simulink model "MODEL_joy"  (R2021a)
settings: Solver=VariableStepAuto  StartTime=0.0  StopTime=inf  RelTol=1e-3
undefined symbols (not defined in the file or in its folder): aircraft, Earth, FandM, MAV, plotprob, u_trim, WGS84
libraries: aerolibfltsims x2, aerolibanimutils x1, aerolibtransform2 x1
settings Model: Creator=DELL  LastModifiedBy=DELL

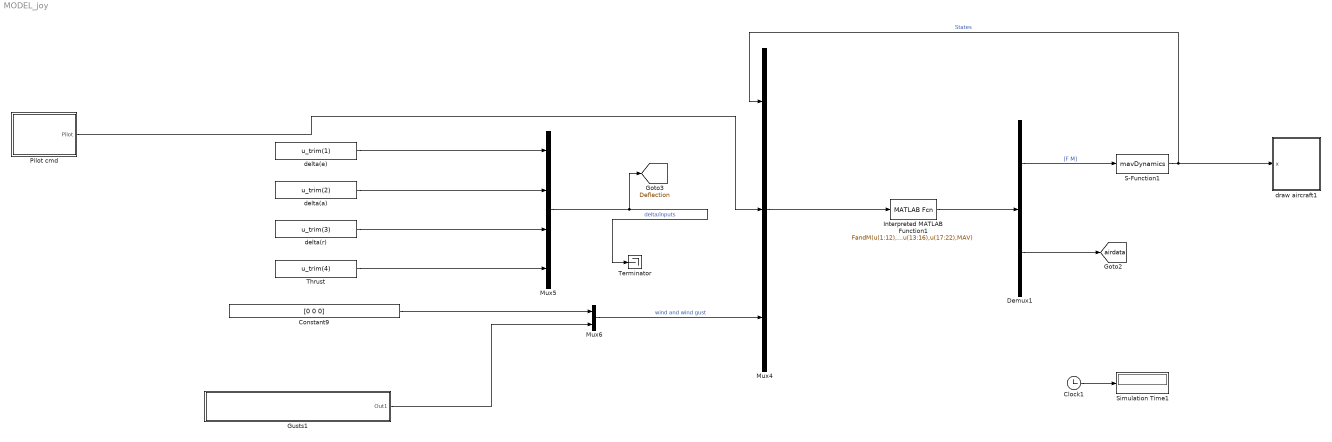
== system MODEL_joy ==
  Clock1 : Clock
  Constant9 : Constant  Value=[0 0 0]
  Demux1 : Demux  Outputs=[6;6]
  Gusts1 : Subsystem
  Interpreted MATLAB Function1 : MATLABFcn  MATLABFcn=FandM(u(1:12),u(13:16),u(17:22),MAV)  OutputDimensions=12
  Mux4 : Mux  Inputs=3
  Mux5 : Mux
  Mux6 : Mux  Inputs=2
  Pilot cmd : Subsystem
  S-Function1 : S-Function  FunctionName=mavDynamics  Parameters=MAV  SFunctionDeploymentMode=off  EnableBusSupport=off
  Simulation Time1 : Display
  Terminator : Terminator
  Thrust : Constant  Value=u_trim(4)
  delta(a) : Constant  Value=u_trim(2)
  delta(e) : Constant  Value=u_trim(1)
  delta(r) : Constant  Value=u_trim(3)
  draw aircraft1 : Subsystem
  tag scope: Deflection=global, airdata=global
  wires:
  Mux6/1 -> Mux4/3  "wind and wind gust"
  Demux1/2 -> [airdata]
  Constant9/1 -> Mux6/1
  Mux5/1 -> Terminator/1, [Deflection]  "delta/inputs"
  Clock1/1 -> Simulation Time1/1
  Mux4/1 -> Interpreted MATLAB Function1/1
  Interpreted MATLAB Function1/1 -> Demux1/1
  S-Function1/1 -> draw aircraft1/1(x), Mux4/1  "States"
  Gusts1/1(Out1) -> Mux6/2
  Demux1/1 -> S-Function1/1  "[F M]"
  delta(e)/1 -> Mux5/1
  delta(a)/1 -> Mux5/2
  delta(r)/1 -> Mux5/3
  Thrust/1 -> Mux5/4
  Pilot cmd/1(Pilot) -> Mux4/2

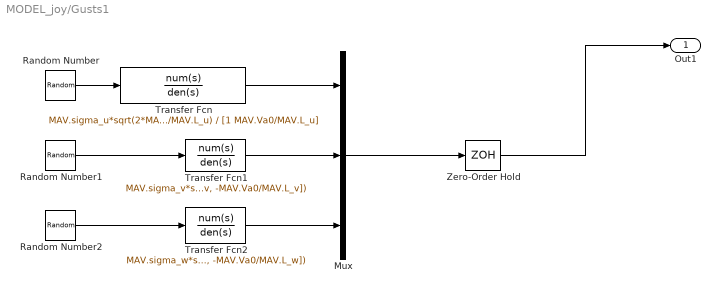
== system MODEL_joy/Gusts1 ==
  Mux : Mux  Inputs=3
  Random Number : RandomNumber  SampleTime=0.1
  Random Number1 : RandomNumber  SampleTime=0.1
  Random Number2 : RandomNumber  SampleTime=0.1
  Transfer Fcn : TransferFcn  Numerator=MAV.sigma_u*sqrt(2*MAV.Va0/MAV.L_u)  Denominator=[1 MAV.Va0/MAV.L_u]
  Transfer Fcn1 : TransferFcn  Numerator=MAV.sigma_v*sqrt(3*MAV.Va0/MAV.L_u)*[0, 1, MAV.Va0/sqrt(3)/MAV.L_v]  Denominator=poly([-MAV.Va0/MAV.L_v, -MAV.Va0/MAV.L_v])
  Transfer Fcn2 : TransferFcn  Numerator=MAV.sigma_w*sqrt(3*MAV.Va0/MAV.L_u)*[0, 1, MAV.Va0/sqrt(3)/MAV.L_w]  Denominator=poly([-MAV.Va0/MAV.L_w, -MAV.Va0/MAV.L_w])
  Zero-Order Hold : ZeroOrderHold  SampleTime=-1
  Out1 : Outport
  wires:
  Zero-Order Hold/1 -> Out1/1
  Transfer Fcn2/1 -> Mux/3
  Random Number1/1 -> Transfer Fcn1/1
  Transfer Fcn/1 -> Mux/1
  Random Number/1 -> Transfer Fcn/1
  Transfer Fcn1/1 -> Mux/2
  Random Number2/1 -> Transfer Fcn2/1
  Mux/1 -> Zero-Order Hold/1

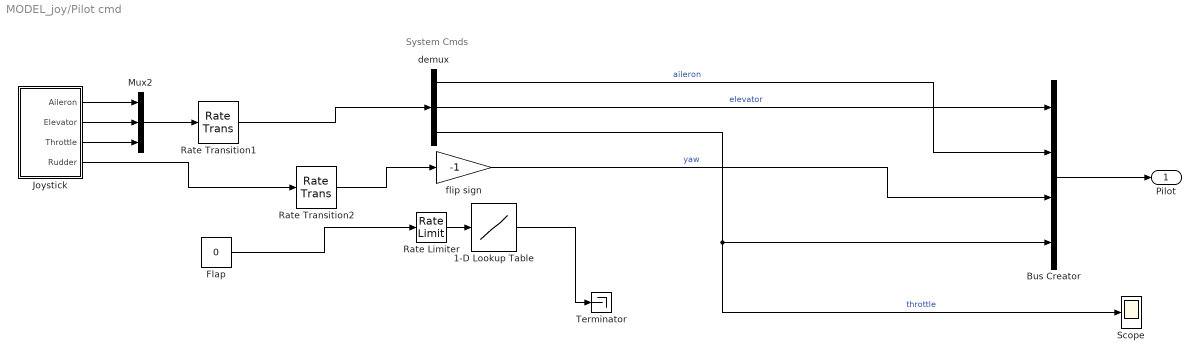
== system MODEL_joy/Pilot cmd ==
  note: System Cmds
  1-D Lookup Table : Lookup_n-D  NumberOfTableDimensions=1  LookupTableObject=''  BreakpointsForDimension1=[0:3]  Table=[0 0 0 0]  SaturateOnIntegerOverflow=on  InputSameDT=on
  Bus Creator : BusCreator  Inputs=4
  Flap : Constant  Value=0
  Joystick : Subsystem
  Mux2 : Mux  Inputs=3
  Rate Limiter : RateLimiter  RisingSlewLimit=0.5  FallingSlewLimit=-0.5
  Rate Transition1 : RateTransition  OutPortSampleTime=0
  Rate Transition2 : RateTransition  OutPortSampleTime=0
  Scope : Scope
  Terminator : Terminator
  demux : Demux  Outputs=3
      settings: DisplayOption=none
  flip sign : Gain  Gain=-1  SaturateOnIntegerOverflow=on  OutDataTypeStr=Inherit: Same as input  ParamDataTypeStr=Inherit: Same as input
  Pilot : Outport  VectorParamsAs1DForOutWhenUnconnected=off
  wires:
  Joystick/1(Aileron) -> Mux2/1
  Joystick/3(Throttle) -> Mux2/3
  Mux2/1 -> Rate Transition1/1
  Joystick/4(Rudder) -> Rate Transition2/1
  Joystick/2(Elevator) -> Mux2/2
  Bus Creator/1 -> Pilot/1
  1-D Lookup Table/1 -> Terminator/1
  demux/2 -> Bus Creator/1  "elevator"
  demux/1 -> Bus Creator/2  "aileron"
  Rate Limiter/1 -> 1-D Lookup Table/1
  Flap/1 -> Rate Limiter/1
  Rate Transition1/1 -> demux/1
  Rate Transition2/1 -> flip sign/1
  flip sign/1 -> Bus Creator/3  "yaw"
  demux/3 -> Scope/1, Bus Creator/4  "throttle"

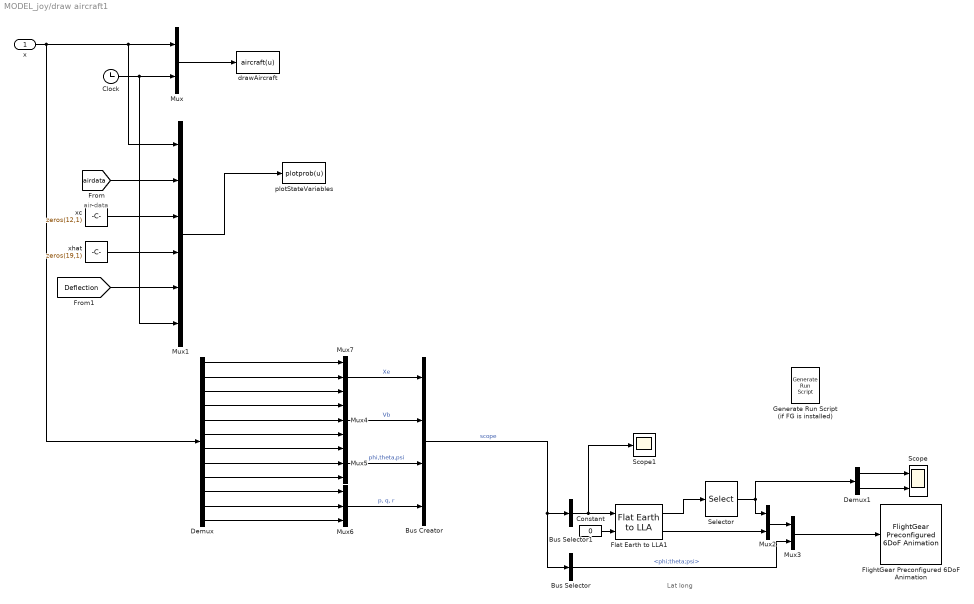
== system MODEL_joy/draw aircraft1 ==
  note: Lat long
  note: air data
  x : Inport
  Bus Creator : BusCreator  Inputs=4
  Bus Selector : BusSelector  OutputSignals=phi;theta;psi
  Bus Selector1 : BusSelector  OutputSignals=Xe  OutputAsBus=on
  Clock : Clock
  Constant : Constant  Value=0
  Demux : Demux  Outputs=12
  Demux1 : Demux  Outputs=2
  Flat Earth to LLA1 : aerolibtransform2/Flat Earth to LLA  units=Metric (MKS)  ptype=Earth (WGS84)  F=1/298.257223563  R=6378137  refPosPort=off  LL0=[37.6272 -122.3896]  psi=0
  FlightGear Preconfigured 6DoF Animation : aerolibfltsims/FlightGear Preconfigured 6DoF Animation  xFlightGearVersion=v2019.1  DestinationIpAddress=127.0.0.1  DestinationPort=5502  SampleTime=1/30  packetVersion=24
  Generate Run Script (if FG is installed) : aerolibfltsims/Generate Run Script  Architecture=Win64  dataFlow=Send  GeometryModelName=c172p  AirportId=KSFO  RunwayId=10L  InitialAltitude=1  InitialHeading=0  OffsetDistance=0  OffsetAzimuth=0  InstallScenery=on  DisableShaders=on  OriginAddress=127.0.0.1  DestinationPort=5502  OriginPort=5505  LocalAddress=127.0.0.1  OutputFileName=runfg_small_UAV.bat  FlightGearBaseDirectory=C:\Program Files\FlightGear 2020.3
  Mux : Mux  Inputs=2
  Mux1 : Mux  Inputs=6
  Mux2 : Mux  Inputs=2
  Mux3 : Mux  Inputs=2
  Mux{4..7} (4 alike) : Mux  Inputs=3
  Scope : Scope  NumInputPorts=2
  Scope1 : Scope
  Selector : Selector  IndexMode=Zero-based  InputPortWidth=2  IndexOptions=Index vector (dialog)  Indices=[1 0]  OutputSizes=1
  drawAircraft : MATLABFcn  MATLABFcn=aircraft(u)  OutputDimensions=0  SampleTime=0.1
  plotStateVariables : MATLABFcn  MATLABFcn=plotprob(u)  OutputDimensions=0  SampleTime=0.1
  xc : Constant  Value=zeros(12,1)
  xhat : Constant  Value=zeros(19,1)
  wires:
  [airdata] -> Mux1/2
  [Deflection] -> Mux1/5
  xc/1 -> Mux1/3
  xhat/1 -> Mux1/4
  Mux1/1 -> plotStateVariables/1
  Clock/1 -> Mux1/6, Mux/2
  x/1 -> Demux/1, Mux1/1, Mux/1
  Mux/1 -> drawAircraft/1
  Demux/1 -> Mux7/1
  Demux/2 -> Mux7/2
  Demux/3 -> Mux7/3
  Mux2/1 -> Mux3/1
  Demux1/2 -> Scope/2
  Flat Earth to LLA1/2 -> Mux2/2
  Bus Selector1/1 -> Flat Earth to LLA1/1, Scope1/1
  Constant/1 -> Flat Earth to LLA1/2
  Bus Selector/1 -> Mux3/2  "<phi;theta;psi>"
  Demux1/1 -> Scope/1
  Flat Earth to LLA1/1 -> Selector/1
  Selector/1 -> Mux2/1, Demux1/1
  Bus Creator/1 -> Bus Selector/1, Bus Selector1/1  "scope"
  Demux/4 -> Mux4/1
  Demux/5 -> Mux4/2
  Demux/6 -> Mux4/3
  Mux4/1 -> Bus Creator/2  "Vb"
  Demux/7 -> Mux5/1
  Demux/8 -> Mux5/2
  Demux/9 -> Mux5/3
  Mux5/1 -> Bus Creator/3  "phi,theta,psi"
  Demux/10 -> Mux6/1
  Demux/11 -> Mux6/2
  Demux/12 -> Mux6/3
  Mux6/1 -> Bus Creator/4  "p, q, r"
  Mux7/1 -> Bus Creator/1  "Xe"
  Mux3/1 -> FlightGear Preconfigured 6DoF Animation/1

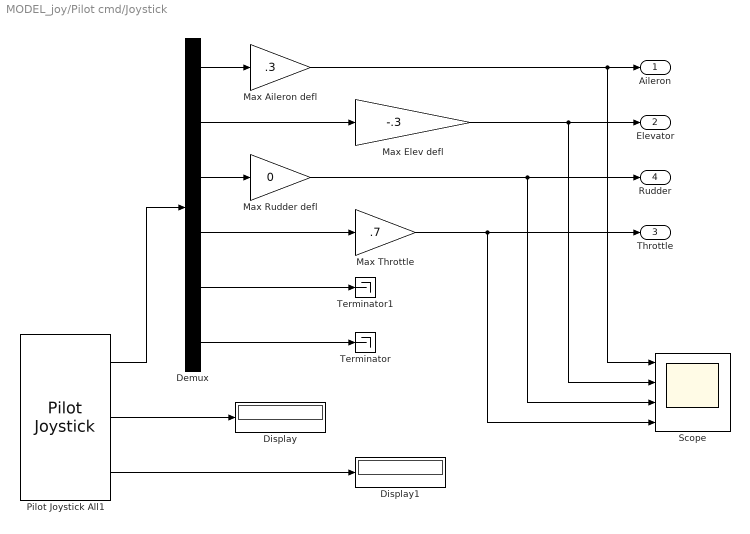
== system MODEL_joy/Pilot cmd/Joystick ==
  Demux : Demux  Outputs=6
  Display : Display
  Display1 : Display
  Max Aileron defl : Gain  Gain=.3
  Max Elev defl : Gain  Gain=-.3
  Max Rudder defl : Gain  Gain=0
  Max Throttle : Gain  Gain=.7
  Pilot Joystick All1 : aerolibanimutils/Pilot Joystick  JoystickID=Joystick1  OutputConfiguration=AllOutputs  SampleTime=1/30
  Scope : Scope  NumInputPorts=4
  Terminator : Terminator
  Terminator1 : Terminator
  Aileron : Outport
  Elevator : Outport  Port=2
  Throttle : Outport  Port=3
  Rudder : Outport  Port=4
  wires:
  Pilot Joystick All1/3 -> Display1/1
  Demux/4 -> Max Throttle/1
  Demux/3 -> Max Rudder defl/1
  Max Aileron defl/1 -> Aileron/1, Scope/1
  Pilot Joystick All1/2 -> Display/1
  Pilot Joystick All1/1 -> Demux/1
  Demux/6 -> Terminator/1
  Demux/5 -> Terminator1/1
  Demux/2 -> Max Elev defl/1
  Demux/1 -> Max Aileron defl/1
  Max Rudder defl/1 -> Scope/3, Rudder/1
  Max Elev defl/1 -> Scope/2, Elevator/1
  Max Throttle/1 -> Scope/4, Throttle/1
